simulink model "W3P1"  (R2020b)
settings: Solver=VariableStepAuto  StartTime=0.0  StopTime=10.0  RelTol=1e-3
settings Model: Creator=saadh  LastModifiedBy=saadh

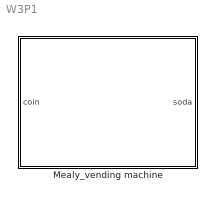
== system W3P1 ==
  Mealy_vending machine : Stateflow chart  TreatAsAtomicUnit=on

== stateflow chart W3P1/Mealy_vending machine ==
  note: The vending machine requires 15 cents to release a can of soda.
      | Nickel=5 cents
      | Dime=10 cents
  state got_0
  state got_nickel
  state got_dime
  (default) -> got_0
  got_0 -> got_nickel [order 1] : [coin==5]{soda=0}
  got_nickel -> got_0 [order 2] : [coin==10]{soda=1}
  got_dime -> got_0 [order 1] : [coin==5]{soda=1}
  got_0 -> got_dime [order 2] : [coin==10]{soda=0}
  got_nickel -> got_dime [order 1] : [coin==5]{soda=0}
  got_dime -> got_nickel [order 2] : [coin==10]{soda=1}
  data: coin input; soda output
